simulink model "full_model_car"  (R2017b)
settings: Solver=ode23s  StartTime=0.0  StopTime=t_max  RelTol=1e-5
undefined symbols (not defined in the file or in its folder): A, Cd, fr, g, lf, lr, m, pp, rho, rw, t_sample, V_F
libraries: simulink x3
settings Model: Creator=João Fernandes  LastModifiedBy=João Fernandes

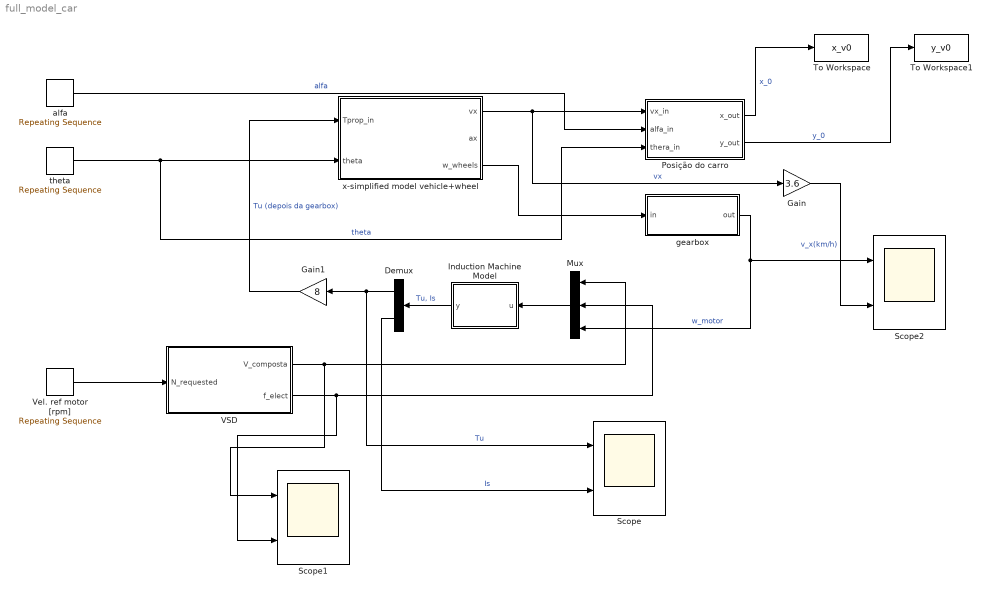
== system full_model_car ==
  Demux : Demux  Outputs=2
  Gain : Gain  Gain=3.6
  Gain1 : Gain  Gain=8
  Induction Machine Model : MATLAB Function  TreatAsAtomicUnit=on
  Mux : Mux  Inputs=3
  Posição do carro : Subsystem
  Scope : Scope  NumInputPorts=2
  Scope1 : Scope  NumInputPorts=2
  Scope2 : Scope  NumInputPorts=2
  To Workspace : ToWorkspace  VariableName=x_v0  SaveFormat=Timeseries  SampleTime=t_sample
  To Workspace1 : ToWorkspace  VariableName=y_v0  SaveFormat=Timeseries  SampleTime=t_sample
  VSD : Subsystem
  Vel. ref motor [rpm] : simulink/Sources/Repeating Sequence  rep_seq_t=v_t  rep_seq_y=v_v
  alfa : simulink/Sources/Repeating Sequence  rep_seq_t=alfa_t  rep_seq_y=alfa_v
  gearbox : Subsystem
  theta : simulink/Sources/Repeating Sequence  rep_seq_t=theta_t  rep_seq_y=theta_v
  x-simplified model vehicle+wheel : Subsystem
  wires:
  x-simplified model vehicle+wheel/1(vx) -> Gain/1, Posição do carro/1(vx_in)  "vx"
  Posição do carro/1(x_out) -> To Workspace/1  "x_0"
  Posição do carro/2(y_out) -> To Workspace1/1  "y_0"
  x-simplified model vehicle+wheel/3(w_wheels) -> gearbox/1(in)
  Mux/1 -> Induction Machine Model/1(u)
  gearbox/1(out) -> Scope2/1, Mux/3  "w_motor"
  Induction Machine Model/1(y) -> Demux/1  "Tu, Is"
  Vel. ref motor [rpm]/1 -> VSD/1(N_requested)
  VSD/1(V_composta) -> Scope1/1, Mux/1
  VSD/2(f_elect) -> Scope1/2, Mux/2
  theta/1 -> x-simplified model vehicle+wheel/2(theta), Posição do carro/3(thera_in)  "theta"
  Demux/1 -> Scope/1, Gain1/1  "Tu"
  alfa/1 -> Posição do carro/2(alfa_in)  "alfa"
  Demux/2 -> Scope/2  "Is"
  Gain/1 -> Scope2/2  "v_x(km/h)"
  Gain1/1 -> x-simplified model vehicle+wheel/1(Tprop_in)  "Tu (depois da gearbox)"

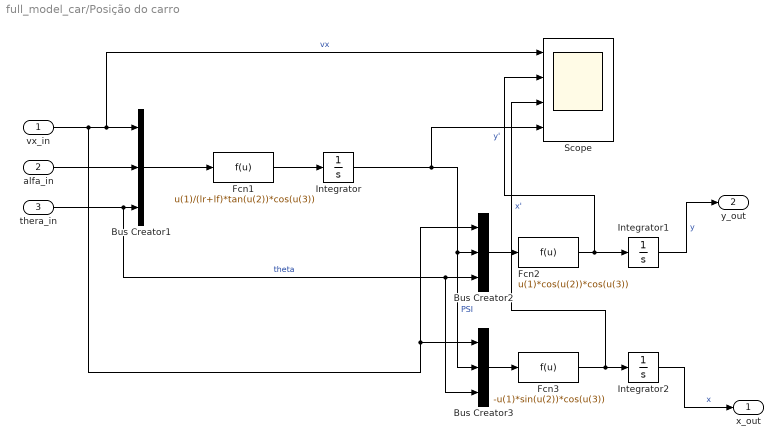
== system full_model_car/Posição do carro ==
  vx_in : Inport
  alfa_in : Inport  Port=2
  thera_in : Inport  Port=3
  Bus Creator1 : BusCreator  Inputs=3
  Bus Creator2 : BusCreator  Inputs=3
  Bus Creator3 : BusCreator  Inputs=3
  Fcn1 : Fcn  Expr=u(1)/(lr+lf)*tan(u(2))*cos(u(3))
  Fcn2 : Fcn  Expr=u(1)*cos(u(2))*cos(u(3))
  Fcn3 : Fcn  Expr=-u(1)*sin(u(2))*cos(u(3))
  Integrator : Integrator
  Integrator1 : Integrator
  Integrator2 : Integrator
  Scope : Scope  NumInputPorts=4
  x_out : Outport
  y_out : Outport  Port=2
  wires:
  Integrator1/1 -> y_out/1  "y"
  Integrator2/1 -> x_out/1  "x"
  thera_in/1 -> Bus Creator3/3, Bus Creator2/3, Bus Creator1/3  "theta"
  Bus Creator1/1 -> Fcn1/1
  Fcn1/1 -> Integrator/1
  Bus Creator2/1 -> Fcn2/1
  vx_in/1 -> Bus Creator2/1, Bus Creator3/1, Scope/1, Bus Creator1/1  "vx"
  Fcn2/1 -> Scope/2, Integrator1/1  "y'"
  Fcn3/1 -> Scope/3, Integrator2/1  "x'"
  Integrator/1 -> Scope/4, Bus Creator3/2, Bus Creator2/2  "PSI"
  Bus Creator3/1 -> Fcn3/1
  alfa_in/1 -> Bus Creator1/2

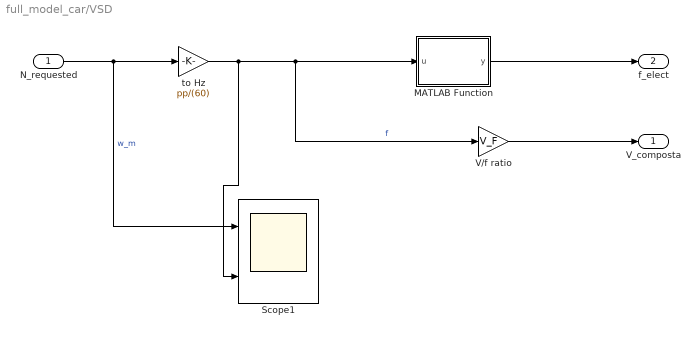
== system full_model_car/VSD ==
  N_requested : Inport
  MATLAB Function : MATLAB Function  TreatAsAtomicUnit=on
  Scope1 : Scope  NumInputPorts=2
  V/f ratio : Gain  Gain=V_F
  to Hz : Gain  Gain=pp/(60)
  V_composta : Outport
  f_elect : Outport  Port=2
  wires:
  N_requested/1 -> Scope1/1, to Hz/1  "w_m"
  to Hz/1 -> V/f ratio/1, MATLAB Function/1(u), Scope1/2  "f"
  MATLAB Function/1(y) -> f_elect/1
  V/f ratio/1 -> V_composta/1

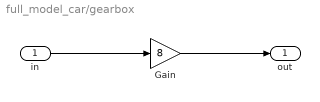
== system full_model_car/gearbox ==
  in : Inport
  Gain : Gain  Gain=8
  out : Outport
  wires:
  in/1 -> Gain/1
  Gain/1 -> out/1

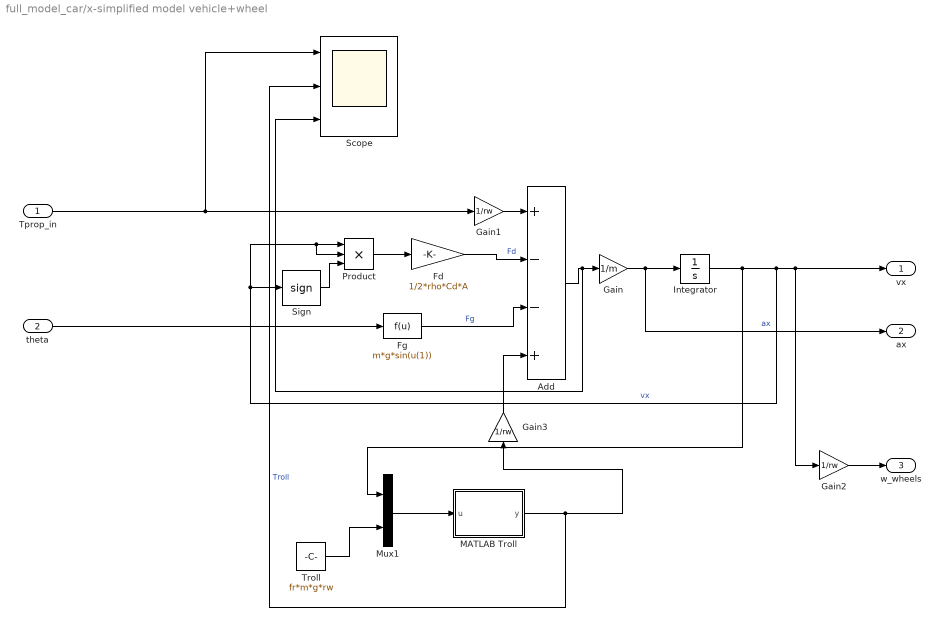
== system full_model_car/x-simplified model vehicle+wheel ==
  Tprop_in : Inport
  theta : Inport  Port=2
  Add : Sum  Inputs=+--+
  Fd : Gain  Gain=1/2*rho*Cd*A
  Fg : Fcn  Expr=m*g*sin(u(1))
  Gain : Gain  Gain=1/m
  Gain1 : Gain  Gain=1/rw
  Gain2 : Gain  Gain=1/rw
  Gain3 : Gain  Gain=1/rw
  Integrator : Integrator
  MATLAB Troll : MATLAB Function  TreatAsAtomicUnit=on
  Mux1 : Mux  Inputs=2
  Product : Product  Inputs=3
  Scope : Scope  NumInputPorts=3
  Sign : Signum
  "Troll " : Constant  Value=fr*m*g*rw
  vx : Outport
  ax : Outport  Port=2
  w_wheels : Outport  Port=3
  wires:
  Product/1 -> Fd/1
  theta/1 -> Fg/1
  Fg/1 -> Add/3  "Fg"
  Add/1 -> Scope/3, Gain/1
  Gain/1 -> Integrator/1, ax/1  "ax"
  Fd/1 -> Add/2  "Fd"
  Integrator/1 -> Mux1/1, Gain2/1, vx/1, Sign/1, Product/2, Product/1  "vx"
  Sign/1 -> Product/3
  Gain1/1 -> Add/1
  Gain2/1 -> w_wheels/1
  Tprop_in/1 -> Scope/1, Gain1/1
  "Troll "/1 -> Mux1/2
  Mux1/1 -> MATLAB Troll/1(u)
  MATLAB Troll/1(y) -> Scope/2, Gain3/1  "Troll"
  Gain3/1 -> Add/4

== matlab function full_model_car/x-simplified model vehicle+wheel/MATLAB Troll ==
  data: u input; y output
function y = fTout(u)
y=0;
vx=u(1);
Troll=u(2);

if vx>0.01
   y=-Troll; % se o carro estiver a andar para a frente, este atrito trava o movimento
elseif vx<-0.01
    y=Troll; % se o carro estiver a andar para trás, este atrito trava o movimento
else
    y=0;
end

== matlab function full_model_car/Induction Machine Model ==
  data: u input; y output
function y = IMmodel(u)
y=[0 0];
% entradas: 
% u(1) - tensão composta
% u(2) - frequência elétrica
% u(3) - velocidade de rotação do motor em rad/s

% saida
% y(1) - torque_util
% y(2) - corrente do estator

% dados do motor de indução
pp=2;
Rs=8.56e-3;
Ls=0.06292e-3;
Lm=1.01220e-3;
Rr=5.10e-3;
Lr=0.06709e-3;   

V=u(1)/sqrt(3); % tensão simples [V]
f=u(2); % frequência elétrica [Hz] - input do controlador V/f 
w=2*pi*f; % velocidade elétrica angular [rad/s]
Ws=w/pp; % Velocidade do campo girante [rad/s]
Wr=u(3); % Velocidade de rotação do motor [rad/s]
s=(Ws-Wr)/Ws;

% modelo do motor
Zs=Rs+1i*w*Ls;
Zr1=Rr+1i*w*Lr;
Zr2=Rr*(1-s)/s;
Zr=Zr1+Zr2;
Zm=1i*w*Lm;

% Correntes
Is=V/(Zs+Zr*Zm/(Zr+Zm)); % corrente no estator [A]
Um=V-Zs*Is; % tensão de magnetização [V]
Ir=Um/(Zr); % corrente no rotor [A]
Im=Um/Zm; % corrente de magnetização [A]

% potência mecânica:
% Pm=3*Zr2*abs(Ir)^2;
if Wr==Ws
    Tu=0;
else
    Tu=(3*Rr*abs(Ir)^2)/(s*Ws);
end

% output é o Tu e Is.
y(1) = Tu;
y(2) = abs(Is);

== matlab function full_model_car/VSD/MATLAB Function ==
  data: u input; y output
function y = f_not_zero(u)
y=0;


if u==0
    y=0.001;
else
    y=u;
end
